simulink model "Controller_ABS_VLC_AYC"  (Simulink 8.7)
settings: Solver=ode3  SolverMode=SingleTasking  StartTime=0.0  StopTime=6  FixedStep=0.001  RelTol=1e-3
undefined symbols (not defined in the file): fdesignblkfcn, gcbh, Lf, Lr, T_Avail
libraries: fuzblock x17, simulink x8
(part 1 of 2)
settings Model: MinMaxOverflowLogging=ForceOff  Creator=MR Spyder  LastModifiedBy=kschmutz
settings DataIOCC: SignalLoggingSaveFormat=ModelDataLogs  SaveOutput=off  SaveTime=off
settings OptimizationCC: DefaultParameterBehavior=Inlined  ExpressionDepthLimit=2147483647
settings DebuggingCC: SolverPrmCheckMsg=warning  FcnCallInpInsideContextMsg=EnableAllAsWarning  StateNameClashWarn=warning
settings GRTTargetCC: CombineOutputUpdateFcns=off  GRTInterface=on

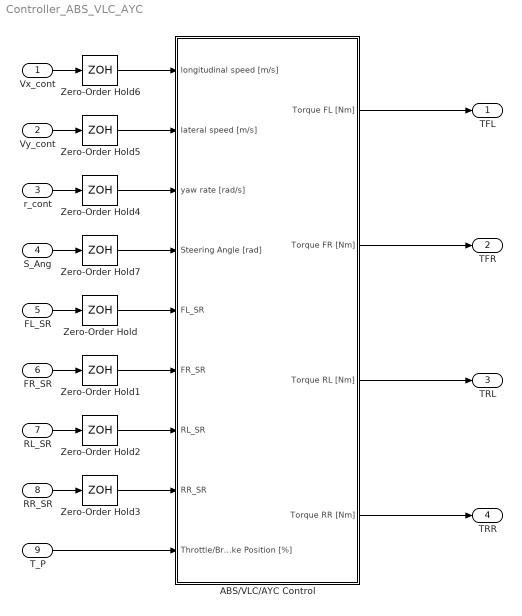
== system Controller_ABS_VLC_AYC ==
  Vx_cont : Inport
  Vy_cont : Inport  Port=2
  r_cont : Inport  Port=3
  S_Ang : Inport  Port=4
  FL_SR : Inport  Port=5
  FR_SR : Inport  Port=6
  RL_SR : Inport  Port=7
  RR_SR : Inport  Port=8
  T_P : Inport  Port=9
  ABS/VLC/AYC Control : Subsystem
  Zero-Order Hold{,1..7} (8 alike) : ZeroOrderHold  SampleTime=0.001
  TFL : Outport
  TFR : Outport  Port=2
  TRL : Outport  Port=3
  TRR : Outport  Port=4
  wires:
  Vx_cont/1 -> Zero-Order Hold6/1
  Vy_cont/1 -> Zero-Order Hold5/1
  r_cont/1 -> Zero-Order Hold4/1
  S_Ang/1 -> Zero-Order Hold7/1
  FL_SR/1 -> Zero-Order Hold/1
  FR_SR/1 -> Zero-Order Hold1/1
  RL_SR/1 -> Zero-Order Hold2/1
  RR_SR/1 -> Zero-Order Hold3/1
  T_P/1 -> ABS/VLC/AYC Control/9(Throttle/Brake Position [%])
  ABS/VLC/AYC Control/1(Torque FL [Nm]) -> TFL/1
  ABS/VLC/AYC Control/2(Torque FR [Nm]) -> TFR/1
  ABS/VLC/AYC Control/3(Torque RL [Nm]) -> TRL/1
  ABS/VLC/AYC Control/4(Torque RR [Nm]) -> TRR/1
  Zero-Order Hold/1 -> ABS/VLC/AYC Control/5(FL_SR)
  Zero-Order Hold1/1 -> ABS/VLC/AYC Control/6(FR_SR)
  Zero-Order Hold2/1 -> ABS/VLC/AYC Control/7(RL_SR)
  Zero-Order Hold3/1 -> ABS/VLC/AYC Control/8(RR_SR)
  Zero-Order Hold4/1 -> ABS/VLC/AYC Control/3(yaw rate [rad/s])
  Zero-Order Hold5/1 -> ABS/VLC/AYC Control/2(lateral speed [m/s])
  Zero-Order Hold6/1 -> ABS/VLC/AYC Control/1(longitudinal speed [m/s])
  Zero-Order Hold7/1 -> ABS/VLC/AYC Control/4(Steering Angle [rad])

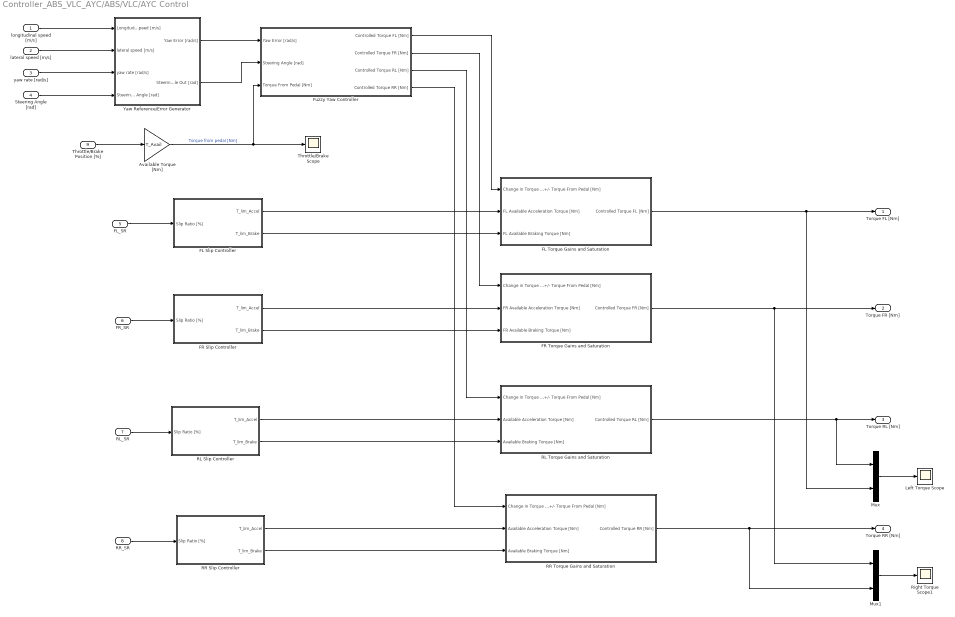
== system Controller_ABS_VLC_AYC/ABS/VLC/AYC Control ==
  longitudinal speed [m/s] : Inport
  lateral speed [m/s] : Inport  Port=2
  yaw rate [rad/s] : Inport  Port=3
  Steering Angle [rad] : Inport  Port=4
  FL_SR : Inport  Port=5
  FR_SR : Inport  Port=6
  RL_SR : Inport  Port=7
  RR_SR : Inport  Port=8
  Throttle/Brake Position [%] : Inport  Port=9
  Available Torque [Nm] : Gain  Gain=T_Avail
  FL Slip Controller : Subsystem
  FL Torque Gains and Saturation : Subsystem
  FR Slip Controller : Subsystem
  FR Torque Gains and Saturation : Subsystem
  Fuzzy Yaw Controller : Subsystem
  Left Torque Scope : Scope
  Mux : Mux  Inputs=2
  Mux1 : Mux  Inputs=2
  RL Slip Controller : Subsystem
  RL Torque Gains and Saturation : Subsystem
  RR Slip Controller : Subsystem
  RR Torque Gains and Saturation : Subsystem
  Right Torque Scope1 : Scope
  Throttle/Brake Scope : Scope
  Yaw Reference/Error Generator : Subsystem
  Torque FL [Nm] : Outport
  Torque FR [Nm] : Outport  Port=2
  Torque RL [Nm] : Outport  Port=3
  Torque RR [Nm] : Outport  Port=4
  wires:
  FL_SR/1 -> FL Slip Controller/1(Slip Ratio [%])
  Mux/1 -> Left Torque Scope/1
  longitudinal speed [m/s]/1 -> Yaw Reference/Error Generator/1(Longitudinal Speed [m/s])
  lateral speed [m/s]/1 -> Yaw Reference/Error Generator/2(lateral speed [m/s])
  yaw rate [rad/s]/1 -> Yaw Reference/Error Generator/3(yaw rate [rad/s])
  Steering Angle [rad]/1 -> Yaw Reference/Error Generator/4(Steering Angle [rad])
  Throttle/Brake Position [%]/1 -> Available Torque [Nm]/1
  Available Torque [Nm]/1 -> Fuzzy Yaw Controller/3(Torque From Pedal [Nm]), Throttle/Brake Scope/1  "Torque from pedal [Nm]"
  FL Slip Controller/1(T_lim_Accel) -> FL Torque Gains and Saturation/2(FL Available Acceleration Torque [Nm])
  FL Slip Controller/2(T_lim_Brake) -> FL Torque Gains and Saturation/3(FL Available Braking Torque [Nm])
  Yaw Reference/Error Generator/1(Yaw Error [rad/s]) -> Fuzzy Yaw Controller/1(Yaw Error [rad/s])
  Yaw Reference/Error Generator/2(Steering Angle Out [rad]) -> Fuzzy Yaw Controller/2(Steering Angle [rad])
  Fuzzy Yaw Controller/1(Controlled Torque FL [Nm]) -> FL Torque Gains and Saturation/1(Change in Torque +/- Torque From Pedal [Nm])
  Fuzzy Yaw Controller/2(Controlled Torque FR [Nm]) -> FR Torque Gains and Saturation/1(Change in Torque +/- Torque From Pedal [Nm])
  Fuzzy Yaw Controller/3(Controlled Torque RL [Nm]) -> RL Torque Gains and Saturation/1(Change in Torque +/- Torque From Pedal [Nm])
  Fuzzy Yaw Controller/4(Controlled Torque RR [Nm]) -> RR Torque Gains and Saturation/1(Change in Torque +/- Torque From Pedal [Nm])
  FL Torque Gains and Saturation/1(Controlled Torque FL [Nm]) -> Torque FL [Nm]/1, Mux/2
  FR Torque Gains and Saturation/1(Controlled Torque FR [Nm]) -> Torque FR [Nm]/1, Mux1/1
  RL Torque Gains and Saturation/1(Controlled Torque RL [Nm]) -> Torque RL [Nm]/1, Mux/1
  RR Torque Gains and Saturation/1(Controlled Torque RR [Nm]) -> Torque RR [Nm]/1, Mux1/2
  RL_SR/1 -> RL Slip Controller/1(Slip Ratio [%])
  RR_SR/1 -> RR Slip Controller/1(Slip Ratio [%])
  FR Slip Controller/1(T_lim_Accel) -> FR Torque Gains and Saturation/2(FR Available Acceleration Torque [Nm])
  FR Slip Controller/2(T_lim_Brake) -> FR Torque Gains and Saturation/3(FR Available Braking Torque [Nm])
  RL Slip Controller/1(T_lim_Accel) -> RL Torque Gains and Saturation/2(Available Acceleration Torque [Nm])
  RL Slip Controller/2(T_lim_Brake) -> RL Torque Gains and Saturation/3(Available Braking Torque [Nm])
  RR Slip Controller/1(T_lim_Accel) -> RR Torque Gains and Saturation/2(Available Acceleration Torque [Nm])
  RR Slip Controller/2(T_lim_Brake) -> RR Torque Gains and Saturation/3(Available Braking Torque [Nm])
  Mux1/1 -> Right Torque Scope1/1
  FR_SR/1 -> FR Slip Controller/1(Slip Ratio [%])

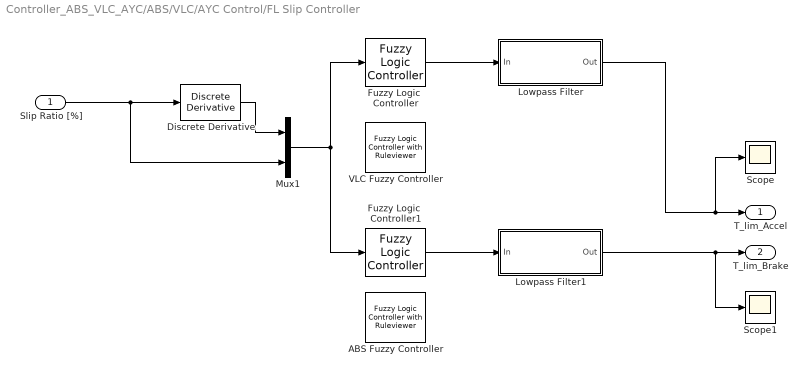
== system Controller_ABS_VLC_AYC/ABS/VLC/AYC Control/FL Slip Controller ==
  Slip Ratio [%] : Inport
  ABS Fuzzy Controller : fuzblock/Fuzzy Logic  Controller  with Ruleviewer  fismatrix=Fuzzy_Slip_Ctl_ABS  Ts=.1
  Discrete Derivative : simulink/Discrete/Discrete Derivative  gainval=1.0  ICPrevScaledInput=0.0  InputProcessing=Inherited  OutMin=[]  OutMax=[]  OutDataType=fixdt(1, 16)  OutScaling=2^-10  DoSatur=off
  Fuzzy Logic  Controller : fuzblock/Fuzzy Logic  Controller  fis=Fuzzy_Slip_Ctl_VLC
  Fuzzy Logic  Controller1 : fuzblock/Fuzzy Logic  Controller  fis=Fuzzy_Slip_Ctl_ABS
  Lowpass Filter : Subsystem  DialogController=fdesignblkfcn  DialogControllerArgs=DataTag1  InitFcn=fdesignblkfcn(gcbh, {'InitFcn'});  mask(Lowpass Filter){}
      mask help: Design a lowpass filter
      settings: CopyFcn=fdesignblkfcn(gcbh, {'CopyFcn'});
      mask Help: helpview(mapfilelocation('dsp'), 'dsplowpassfilter');
      mask Display: disp('Lowpass')
  Lowpass Filter1 : Subsystem  DialogController=fdesignblkfcn  DialogControllerArgs=DataTag3  InitFcn=fdesignblkfcn(gcbh, {'InitFcn'});  mask(Lowpass Filter){}
      mask help: Design a lowpass filter
      settings: CopyFcn=fdesignblkfcn(gcbh, {'CopyFcn'});
      mask Help: helpview(mapfilelocation('dsp'), 'dsplowpassfilter');
      mask Display: disp('Lowpass')
  Mux1 : Mux  Inputs=2
  Scope : Scope
  Scope1 : Scope
  VLC Fuzzy Controller : fuzblock/Fuzzy Logic  Controller  with Ruleviewer  fismatrix=Fuzzy_Slip_Ctl_VLC  Ts=.1
  T_lim_Accel : Outport
  T_lim_Brake : Outport  Port=2
  wires:
  Mux1/1 -> Fuzzy Logic  Controller/1, Fuzzy Logic  Controller1/1
  Slip Ratio [%]/1 -> Mux1/2, Discrete Derivative/1
  Discrete Derivative/1 -> Mux1/1
  Fuzzy Logic  Controller/1 -> Lowpass Filter/1(In)
  Fuzzy Logic  Controller1/1 -> Lowpass Filter1/1(In)
  Lowpass Filter/1(Out) -> T_lim_Accel/1, Scope/1
  Lowpass Filter1/1(Out) -> T_lim_Brake/1, Scope1/1

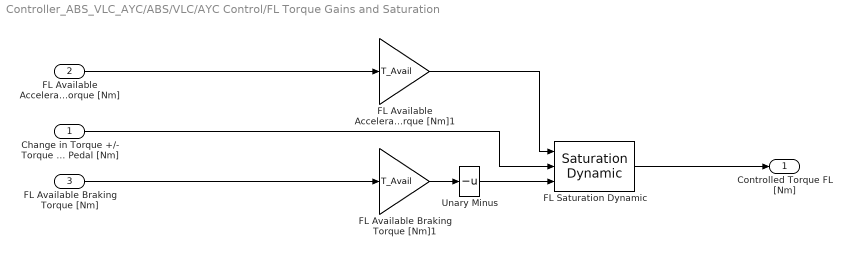
== system Controller_ABS_VLC_AYC/ABS/VLC/AYC Control/FL Torque Gains and Saturation ==
  Change in Torque +/- Torque From Pedal [Nm] : Inport
  FL Available Acceleration Torque [Nm] : Inport  Port=2
  FL Available Braking Torque [Nm] : Inport  Port=3
  FL Available Acceleration Torque [Nm]1 : Gain  Gain=T_Avail
  FL Available Braking Torque [Nm]1 : Gain  Gain=T_Avail
  FL Saturation Dynamic : simulink/Discontinuities/Saturation Dynamic  OutMin=[]  OutMax=[]  OutDataTypeStr=Inherit: Same as second input  OutDataType=fixdt(1, 16)  OutScaling=2^-10  DoSatur=off
  Unary Minus : UnaryMinus
  Controlled Torque FL [Nm] : Outport
  wires:
  FL Available Acceleration Torque [Nm]1/1 -> FL Saturation Dynamic/1
  Unary Minus/1 -> FL Saturation Dynamic/3
  FL Available Braking Torque [Nm]1/1 -> Unary Minus/1
  FL Available Acceleration Torque [Nm]/1 -> FL Available Acceleration Torque [Nm]1/1
  FL Available Braking Torque [Nm]/1 -> FL Available Braking Torque [Nm]1/1
  Change in Torque +/- Torque From Pedal [Nm]/1 -> FL Saturation Dynamic/2
  FL Saturation Dynamic/1 -> Controlled Torque FL [Nm]/1

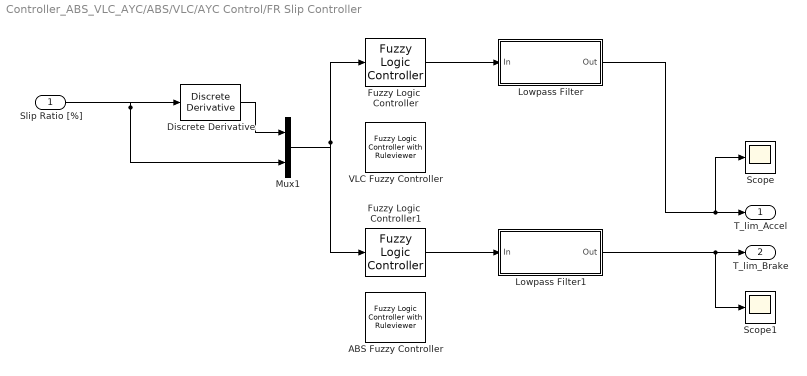
== system Controller_ABS_VLC_AYC/ABS/VLC/AYC Control/FR Slip Controller ==
  Slip Ratio [%] : Inport
  ABS Fuzzy Controller : fuzblock/Fuzzy Logic  Controller  with Ruleviewer  fismatrix=Fuzzy_Slip_Ctl_ABS  Ts=.1
  Discrete Derivative : simulink/Discrete/Discrete Derivative  gainval=1.0  ICPrevScaledInput=0.0  InputProcessing=Inherited  OutMin=[]  OutMax=[]  OutDataType=fixdt(1, 16)  OutScaling=2^-10  DoSatur=off
  Fuzzy Logic  Controller : fuzblock/Fuzzy Logic  Controller  fis=Fuzzy_Slip_Ctl_VLC
  Fuzzy Logic  Controller1 : fuzblock/Fuzzy Logic  Controller  fis=Fuzzy_Slip_Ctl_ABS
  Lowpass Filter : Subsystem  DialogController=fdesignblkfcn  DialogControllerArgs=DataTag5  InitFcn=fdesignblkfcn(gcbh, {'InitFcn'});  mask(Lowpass Filter){}
      mask help: Design a lowpass filter
      settings: CopyFcn=fdesignblkfcn(gcbh, {'CopyFcn'});
      mask Help: helpview(mapfilelocation('dsp'), 'dsplowpassfilter');
      mask Display: disp('Lowpass')
  Lowpass Filter1 : Subsystem  DialogController=fdesignblkfcn  DialogControllerArgs=DataTag7  InitFcn=fdesignblkfcn(gcbh, {'InitFcn'});  mask(Lowpass Filter){}
      mask help: Design a lowpass filter
      settings: CopyFcn=fdesignblkfcn(gcbh, {'CopyFcn'});
      mask Help: helpview(mapfilelocation('dsp'), 'dsplowpassfilter');
      mask Display: disp('Lowpass')
  Mux1 : Mux  Inputs=2
  Scope : Scope
  Scope1 : Scope
  VLC Fuzzy Controller : fuzblock/Fuzzy Logic  Controller  with Ruleviewer  fismatrix=Fuzzy_Slip_Ctl_VLC  Ts=.1
  T_lim_Accel : Outport
  T_lim_Brake : Outport  Port=2
  wires:
  Mux1/1 -> Fuzzy Logic  Controller/1, Fuzzy Logic  Controller1/1
  Slip Ratio [%]/1 -> Mux1/2, Discrete Derivative/1
  Discrete Derivative/1 -> Mux1/1
  Fuzzy Logic  Controller/1 -> Lowpass Filter/1(In)
  Fuzzy Logic  Controller1/1 -> Lowpass Filter1/1(In)
  Lowpass Filter/1(Out) -> T_lim_Accel/1, Scope/1
  Lowpass Filter1/1(Out) -> T_lim_Brake/1, Scope1/1

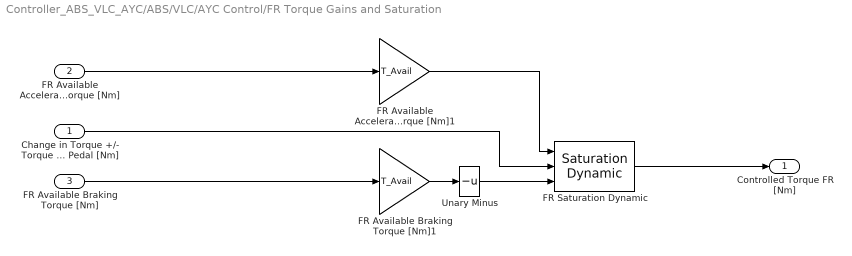
== system Controller_ABS_VLC_AYC/ABS/VLC/AYC Control/FR Torque Gains and Saturation ==
  Change in Torque +/- Torque From Pedal [Nm] : Inport
  FR Available Acceleration Torque [Nm] : Inport  Port=2
  FR Available Braking Torque [Nm] : Inport  Port=3
  FR Available Acceleration Torque [Nm]1 : Gain  Gain=T_Avail
  FR Available Braking Torque [Nm]1 : Gain  Gain=T_Avail
  FR Saturation Dynamic : simulink/Discontinuities/Saturation Dynamic  OutMin=[]  OutMax=[]  OutDataTypeStr=Inherit: Same as second input  OutDataType=fixdt(1, 16)  OutScaling=2^-10  DoSatur=off
  Unary Minus : UnaryMinus
  Controlled Torque FR [Nm] : Outport
  wires:
  FR Available Acceleration Torque [Nm]1/1 -> FR Saturation Dynamic/1
  Unary Minus/1 -> FR Saturation Dynamic/3
  FR Available Braking Torque [Nm]1/1 -> Unary Minus/1
  FR Available Acceleration Torque [Nm]/1 -> FR Available Acceleration Torque [Nm]1/1
  FR Available Braking Torque [Nm]/1 -> FR Available Braking Torque [Nm]1/1
  Change in Torque +/- Torque From Pedal [Nm]/1 -> FR Saturation Dynamic/2
  FR Saturation Dynamic/1 -> Controlled Torque FR [Nm]/1

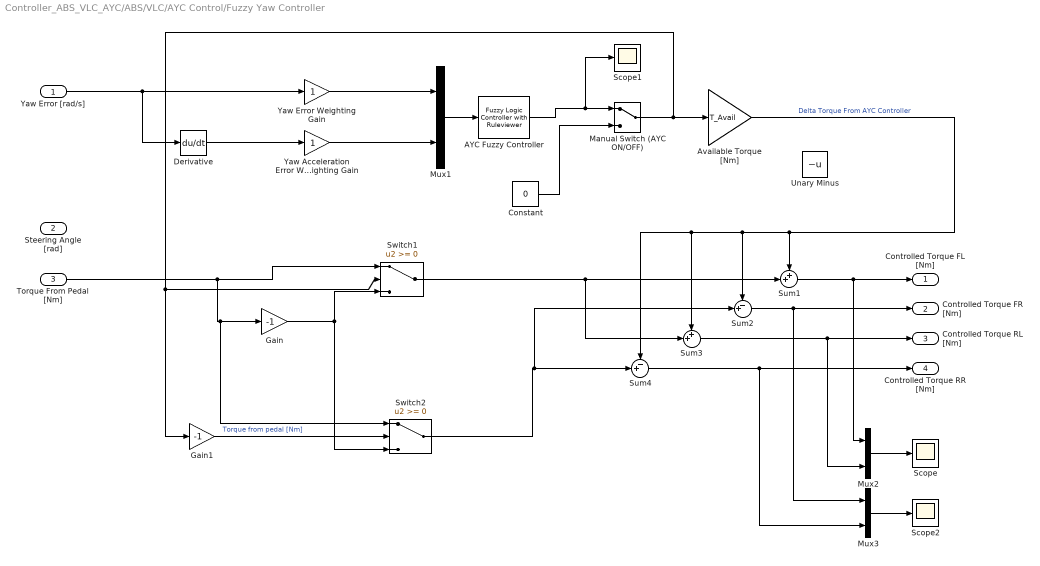
== system Controller_ABS_VLC_AYC/ABS/VLC/AYC Control/Fuzzy Yaw Controller ==
  Yaw Error [rad/s] : Inport
  Steering Angle [rad] : Inport  Port=2
  Torque From Pedal [Nm] : Inport  Port=3
  AYC Fuzzy Controller : fuzblock/Fuzzy Logic  Controller  with Ruleviewer  fismatrix=Fuzzy_AYC_Ctl  Ts=.1
  Available Torque [Nm] : Gain  Gain=T_Avail
  Constant : Constant  Value=0
  Derivative : Derivative
  Gain : Gain  Gain=-1
  Gain1 : Gain  Gain=-1
  Manual Switch (AYC ON/OFF) : ManualSwitch
  Mux1 : Mux  Inputs=2
  Mux2 : Mux  Inputs=2
  Mux3 : Mux  Inputs=2
  Scope : Scope
  Scope1 : Scope
  Scope2 : Scope
  Sum1 : Sum  Inputs=++|
  Sum2 : Sum  Inputs=-+|
  Sum3 : Sum  Inputs=++|
  Sum4 : Sum  Inputs=-+|
  Switch1 : Switch
  Switch2 : Switch
  Unary Minus : UnaryMinus
  Yaw Acceleration Error Weighting Gain : Gain
  Yaw Error Weighting Gain : Gain
  Controlled Torque FL [Nm] : Outport
  Controlled Torque FR [Nm] : Outport  Port=2
  Controlled Torque RL [Nm] : Outport  Port=3
  Controlled Torque RR [Nm] : Outport  Port=4
  wires:
  Sum1/1 -> Controlled Torque FL [Nm]/1, Mux2/1
  Sum2/1 -> Controlled Torque FR [Nm]/1, Mux3/1
  Sum3/1 -> Controlled Torque RL [Nm]/1, Mux2/2
  Sum4/1 -> Controlled Torque RR [Nm]/1, Mux3/2
  Mux1/1 -> AYC Fuzzy Controller/1
  Yaw Error [rad/s]/1 -> Yaw Error Weighting Gain/1, Derivative/1
  Yaw Error Weighting Gain/1 -> Mux1/1
  Yaw Acceleration Error Weighting Gain/1 -> Mux1/2
  Mux2/1 -> Scope/1
  AYC Fuzzy Controller/1 -> Manual Switch (AYC ON/OFF)/1, Scope1/1
  Constant/1 -> Manual Switch (AYC ON/OFF)/2
  Manual Switch (AYC ON/OFF)/1 -> Gain1/1, Switch1/2, Available Torque [Nm]/1
  Mux3/1 -> Scope2/1
  Available Torque [Nm]/1 -> Sum4/1, Sum3/1, Sum2/1, Sum1/1  "Delta Torque From AYC Controller"
  Derivative/1 -> Yaw Acceleration Error Weighting Gain/1
  Switch1/1 -> Sum3/2, Sum1/2
  Gain/1 -> Switch2/3, Switch1/3
  Torque From Pedal [Nm]/1 -> Switch2/1, Gain/1, Switch1/1  "Torque from pedal [Nm]"
  Switch2/1 -> Sum2/2, Sum4/2
  Gain1/1 -> Switch2/2

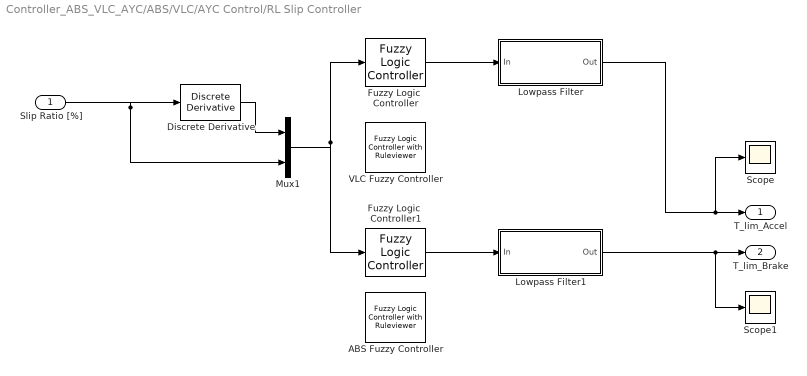
== system Controller_ABS_VLC_AYC/ABS/VLC/AYC Control/RL Slip Controller ==
  Slip Ratio [%] : Inport
  ABS Fuzzy Controller : fuzblock/Fuzzy Logic  Controller  with Ruleviewer  fismatrix=Fuzzy_Slip_Ctl_ABS  Ts=.1
  Discrete Derivative : simulink/Discrete/Discrete Derivative  gainval=1.0  ICPrevScaledInput=0.0  InputProcessing=Inherited  OutMin=[]  OutMax=[]  OutDataType=fixdt(1, 16)  OutScaling=2^-10  DoSatur=off
  Fuzzy Logic  Controller : fuzblock/Fuzzy Logic  Controller  fis=Fuzzy_Slip_Ctl_VLC
  Fuzzy Logic  Controller1 : fuzblock/Fuzzy Logic  Controller  fis=Fuzzy_Slip_Ctl_ABS
  Lowpass Filter : Subsystem  DialogController=fdesignblkfcn  DialogControllerArgs=DataTag9  InitFcn=fdesignblkfcn(gcbh, {'InitFcn'});  mask(Lowpass Filter){}
      mask help: Design a lowpass filter
      settings: CopyFcn=fdesignblkfcn(gcbh, {'CopyFcn'});
      mask Help: helpview(mapfilelocation('dsp'), 'dsplowpassfilter');
      mask Display: disp('Lowpass')
  Lowpass Filter1 : Subsystem  DialogController=fdesignblkfcn  DialogControllerArgs=DataTag11  InitFcn=fdesignblkfcn(gcbh, {'InitFcn'});  mask(Lowpass Filter){}
      mask help: Design a lowpass filter
      settings: CopyFcn=fdesignblkfcn(gcbh, {'CopyFcn'});
      mask Help: helpview(mapfilelocation('dsp'), 'dsplowpassfilter');
      mask Display: disp('Lowpass')
  Mux1 : Mux  Inputs=2
  Scope : Scope
  Scope1 : Scope
  VLC Fuzzy Controller : fuzblock/Fuzzy Logic  Controller  with Ruleviewer  fismatrix=Fuzzy_Slip_Ctl_VLC  Ts=.1
  T_lim_Accel : Outport
  T_lim_Brake : Outport  Port=2
  wires:
  Mux1/1 -> Fuzzy Logic  Controller/1, Fuzzy Logic  Controller1/1
  Slip Ratio [%]/1 -> Mux1/2, Discrete Derivative/1
  Discrete Derivative/1 -> Mux1/1
  Fuzzy Logic  Controller/1 -> Lowpass Filter/1(In)
  Fuzzy Logic  Controller1/1 -> Lowpass Filter1/1(In)
  Lowpass Filter/1(Out) -> T_lim_Accel/1, Scope/1
  Lowpass Filter1/1(Out) -> T_lim_Brake/1, Scope1/1

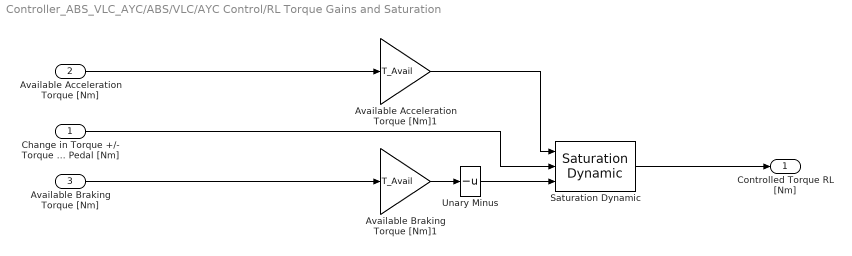
== system Controller_ABS_VLC_AYC/ABS/VLC/AYC Control/RL Torque Gains and Saturation ==
  Change in Torque +/- Torque From Pedal [Nm] : Inport
  Available Acceleration Torque [Nm] : Inport  Port=2
  Available Braking Torque [Nm] : Inport  Port=3
  Available Acceleration Torque [Nm]1 : Gain  Gain=T_Avail
  Available Braking Torque [Nm]1 : Gain  Gain=T_Avail
  Saturation Dynamic : simulink/Discontinuities/Saturation Dynamic  OutMin=[]  OutMax=[]  OutDataTypeStr=Inherit: Same as second input  OutDataType=fixdt(1, 16)  OutScaling=2^-10  DoSatur=off
  Unary Minus : UnaryMinus
  Controlled Torque RL [Nm] : Outport
  wires:
  Available Acceleration Torque [Nm]1/1 -> Saturation Dynamic/1
  Unary Minus/1 -> Saturation Dynamic/3
  Available Braking Torque [Nm]1/1 -> Unary Minus/1
  Available Acceleration Torque [Nm]/1 -> Available Acceleration Torque [Nm]1/1
  Available Braking Torque [Nm]/1 -> Available Braking Torque [Nm]1/1
  Change in Torque +/- Torque From Pedal [Nm]/1 -> Saturation Dynamic/2
  Saturation Dynamic/1 -> Controlled Torque RL [Nm]/1

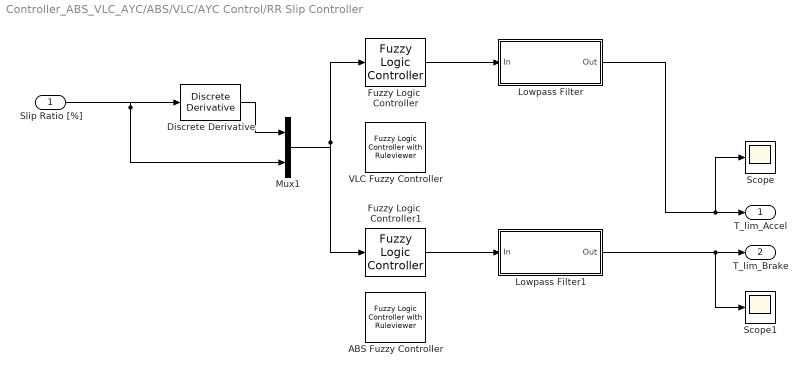
== system Controller_ABS_VLC_AYC/ABS/VLC/AYC Control/RR Slip Controller ==
  Slip Ratio [%] : Inport
  ABS Fuzzy Controller : fuzblock/Fuzzy Logic  Controller  with Ruleviewer  fismatrix=Fuzzy_Slip_Ctl_ABS  Ts=.1
  Discrete Derivative : simulink/Discrete/Discrete Derivative  gainval=1.0  ICPrevScaledInput=0.0  InputProcessing=Inherited  OutMin=[]  OutMax=[]  OutDataType=fixdt(1, 16)  OutScaling=2^-10  DoSatur=off
  Fuzzy Logic  Controller : fuzblock/Fuzzy Logic  Controller  fis=Fuzzy_Slip_Ctl_VLC
  Fuzzy Logic  Controller1 : fuzblock/Fuzzy Logic  Controller  fis=Fuzzy_Slip_Ctl_ABS
  Lowpass Filter : Subsystem  DialogController=fdesignblkfcn  DialogControllerArgs=DataTag13  InitFcn=fdesignblkfcn(gcbh, {'InitFcn'});  mask(Lowpass Filter){}
      mask help: Design a lowpass filter
      settings: CopyFcn=fdesignblkfcn(gcbh, {'CopyFcn'});
      mask Help: helpview(mapfilelocation('dsp'), 'dsplowpassfilter');
      mask Display: disp('Lowpass')
  Lowpass Filter1 : Subsystem  DialogController=fdesignblkfcn  DialogControllerArgs=DataTag15  InitFcn=fdesignblkfcn(gcbh, {'InitFcn'});  mask(Lowpass Filter){}
      mask help: Design a lowpass filter
      settings: CopyFcn=fdesignblkfcn(gcbh, {'CopyFcn'});
      mask Help: helpview(mapfilelocation('dsp'), 'dsplowpassfilter');
      mask Display: disp('Lowpass')
  Mux1 : Mux  Inputs=2
  Scope : Scope
  Scope1 : Scope
  VLC Fuzzy Controller : fuzblock/Fuzzy Logic  Controller  with Ruleviewer  fismatrix=Fuzzy_Slip_Ctl_VLC  Ts=.1
  T_lim_Accel : Outport
  T_lim_Brake : Outport  Port=2
  wires:
  Mux1/1 -> Fuzzy Logic  Controller/1, Fuzzy Logic  Controller1/1
  Slip Ratio [%]/1 -> Mux1/2, Discrete Derivative/1
  Discrete Derivative/1 -> Mux1/1
  Fuzzy Logic  Controller/1 -> Lowpass Filter/1(In)
  Fuzzy Logic  Controller1/1 -> Lowpass Filter1/1(In)
  Lowpass Filter/1(Out) -> T_lim_Accel/1, Scope/1
  Lowpass Filter1/1(Out) -> T_lim_Brake/1, Scope1/1

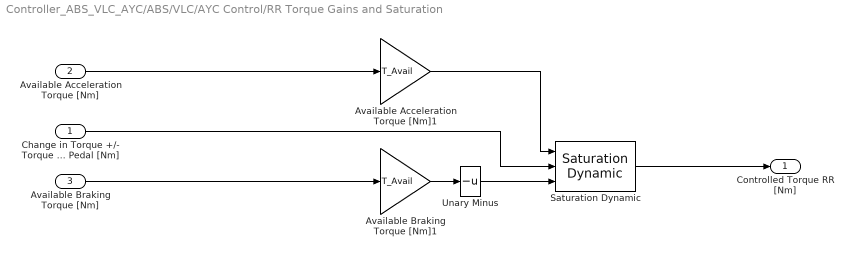
== system Controller_ABS_VLC_AYC/ABS/VLC/AYC Control/RR Torque Gains and Saturation ==
  Change in Torque +/- Torque From Pedal [Nm] : Inport
  Available Acceleration Torque [Nm] : Inport  Port=2
  Available Braking Torque [Nm] : Inport  Port=3
  Available Acceleration Torque [Nm]1 : Gain  Gain=T_Avail
  Available Braking Torque [Nm]1 : Gain  Gain=T_Avail
  Saturation Dynamic : simulink/Discontinuities/Saturation Dynamic  OutMin=[]  OutMax=[]  OutDataTypeStr=Inherit: Same as second input  OutDataType=fixdt(1, 16)  OutScaling=2^-10  DoSatur=off
  Unary Minus : UnaryMinus
  Controlled Torque RR [Nm] : Outport
  wires:
  Available Acceleration Torque [Nm]1/1 -> Saturation Dynamic/1
  Unary Minus/1 -> Saturation Dynamic/3
  Available Braking Torque [Nm]1/1 -> Unary Minus/1
  Available Acceleration Torque [Nm]/1 -> Available Acceleration Torque [Nm]1/1
  Available Braking Torque [Nm]/1 -> Available Braking Torque [Nm]1/1
  Change in Torque +/- Torque From Pedal [Nm]/1 -> Saturation Dynamic/2
  Saturation Dynamic/1 -> Controlled Torque RR [Nm]/1

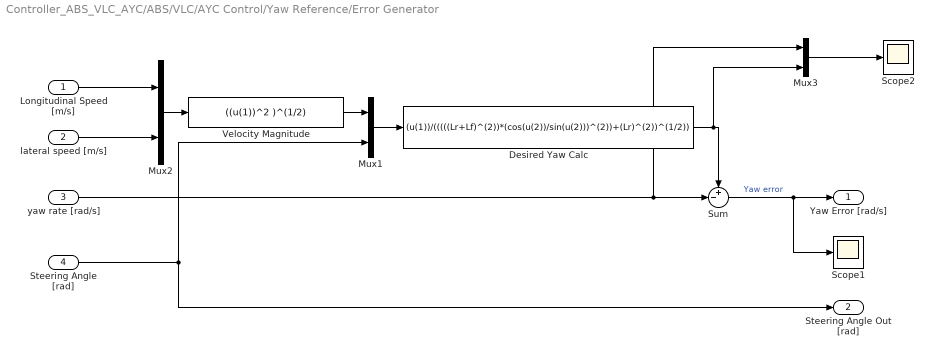
== system Controller_ABS_VLC_AYC/ABS/VLC/AYC Control/Yaw Reference/Error Generator ==
  Longitudinal Speed [m/s] : Inport
  lateral speed [m/s] : Inport  Port=2
  yaw rate [rad/s] : Inport  Port=3
  Steering Angle [rad] : Inport  Port=4
  Desired Yaw Calc : Fcn  Expr=(u(1))/(((((Lr+Lf)^(2))*(cos(u(2))/sin(u(2)))^(2))+(Lr)^(2))^(1/2))
  Mux1 : Mux  Inputs=2
  Mux2 : Mux  Inputs=2
  Mux3 : Mux  Inputs=2
  Scope1 : Scope
  Scope2 : Scope
  Sum : Sum  Inputs=+-|
  Velocity Magnitude : Fcn  Expr=((u(1))^2 )^(1/2)
  Yaw Error [rad/s] : Outport
  Steering Angle Out [rad] : Outport  Port=2
  wires:
  Mux1/1 -> Desired Yaw Calc/1
  lateral speed [m/s]/1 -> Mux2/2
  Longitudinal Speed [m/s]/1 -> Mux2/1
  Mux2/1 -> Velocity Magnitude/1
  Velocity Magnitude/1 -> Mux1/1
  Steering Angle [rad]/1 -> Mux1/2, Steering Angle Out [rad]/1
  yaw rate [rad/s]/1 -> Sum/2, Mux3/1
  Desired Yaw Calc/1 -> Sum/1, Mux3/2
  Sum/1 -> Yaw Error [rad/s]/1, Scope1/1  "Yaw error"
  Mux3/1 -> Scope2/1

== system Controller_ABS_VLC_AYC/ABS/VLC/AYC Control/FL Slip Controller/Lowpass Filter ==
  In : Inport
  Generated Filter Block : DiscreteFir  Tag=BlockMethodSubSystem  Coefficients=[-0.00075646864062919763 -0.00063948505713481811 -0.00086554492949518676 -0.0011037990733813235 -0.001339284284868959 -0.0015547400053551874 -0.0017300944700606284 -0.00184670274387296 -0.0018881302599738493 -0.0018383815937568033 -0.0016908823878034785 -0.0014415887943325673 -0.0010961195158699811 -0.00066631717319359861 -0.00017121409252519941 0.00036359936416717264 0.0009080465739429777 0.0014298736348337699 0.0018960211364896008 0.0022771863603771665 0.0025482618478869408 0.002692222556903226 0.0027008445578628891 0.0025759682427628858 0.0023298680220744062 0.001984391370697888 0.0015692141720698332 0.0011200194544684224 0.00067461876056971635 0.00027061032753731694 -5.866179415617268e-05 -0.00028669635689133085 -0.00039633166387144857 -0.00038148906017572019 -0.0002477702828760265 -1.1936356441557194e-05 0.00029922490683921712 0.00065189802033198212 0.0010079363042756382 0.0013289590517563921 0.0015799187563950311 0.001732598437530234 0.0017685449960751973 0.0016809867202291359 0.001475577844518795 0.0011702671086116819 0.00079334294519489744 0.00038107291302585564 -2.6111427728838237e-05 -0.00038757608995898589 -0.00066664955030768121 -0.00083452345222956249 -0.0008733550143161324 -0.00077824476354573693 -0.00055819296971255797 -0.00023521601512397369 0.00015742126605453337 0.0005785784851626923 0.00098328250386749182 0.0013273087132983671 0.0015718484935428579 0.0016876773286742383 0.0016583648153362584 0.0014824517181836361 0.001173793218361215 0.00076066718725827424 0.00028306324114901494 -0.00021118635508748061 -0.00067122011711513783 -0.0010484581457023382 -0.0013017758532885772 -0.0014019618554660471 -0.0013352201239705105 -0.0011048842486169792 -0.00073165621411404097 -0.00025182527315658872 0.00028610350920870874 0.00082615867146424533 0.0013106234674959305 0.0016860834546990108 0.0019091311706072877 0.0019513306436192534 0.0018025262485976861 0.0014725312016039653 0.00099060478772183152 0.00040292530986260334 -0.00023178098881511844 -0.00084810728175012385 -0.0013806963630004151 -0.0017711026206815544 -0.0019742574925858663 -0.0019635291020280035 -0.0017341538241868613 -0.0013043450108582717 -0.00071404805444023607 -2.1386504594989465e-05 0.00070295843642983579 0.0013828574770577515 0.0019445780369022776 0.0023247321243138005 0.0024772174699799845 0.0023786792654153892 0.0020316457847079574 0.0014650458441179052 0.00073198021892930624 -9.5165616451746313e-05 -0.00093179550640667356 -0.0016896353737900064 -0.002286029399938193 -0.0026528026156592069 -0.0027439824010879752 -0.0025413474050266682 -0.0020572239101028095 -0.0013341713539966283 -0.00044143094406244902 0.00053155699309554165 0.0014839255272411029 0.0023137406585026126 0.0029286981481292974 0.0032562467484617786 0.003251908926443922 0.0029049085085457831 0.0022404564981489922 0.0013182816267311918 0.00022746308219447748 -0.00092196135663783645 -0.0020099732300794516 -0.0029188826132397309 -0.0035458920722500759 -0.0038144882122502053 -0.0036834454103191363 -0.0031524540265802821 -0.0022636032725808913 -0.001098441233437557 0.00022918138522259228 0.0015840095633793522 0.0028228488017388279 0.0038094256961896428 0.0044290486254589569 0.0046015294833341713 0.0042909951378952392 0.0035113829579288443 0.002326900465678434 0.00084726356737852785 -0.00078210688654584614 -0.0023939506744333323 -0.0038159332671489276 -0.0048886091342003283 -0.0054827496552296451 -0.0055142584805278339 -0.0049549620495624256 -0.0038379957384760514 -0.0022570524748253273 -0.00035920054838253909 0.0016681240381698865 0.0036149620582436124 0.0052698289441135563 0.0064418143583644455 0.0069816111699239911 0.0067991979917402107 0.0058762117387505652 0.0042715432406493607 0.0021191551611802598 -0.00038190594776891601 -0.0029847547360424441 -0.0054177398262781288 -0.0074112614644437011 -0.0087258737465600832 -0.0091788423919074678 -0.0086664128929747897 -0.0071793804592940056 -0.004809945117289164 -0.0017488049914463934 0.0017278402015994767 0.0052806440695748677 0.0085371287675241395 ...(+5120 chars)]  InputProcessing=Columns as channels (frame based)
  Out : Outport
  wires:
  In/1 -> Generated Filter Block/1
  Generated Filter Block/1 -> Out/1

== system Controller_ABS_VLC_AYC/ABS/VLC/AYC Control/FL Slip Controller/Lowpass Filter1 ==
  In : Inport
  Generated Filter Block : DiscreteFir  Tag=BlockMethodSubSystem  Coefficients=[-0.00075646864062919763 -0.00063948505713481811 -0.00086554492949518676 -0.0011037990733813235 -0.001339284284868959 -0.0015547400053551874 -0.0017300944700606284 -0.00184670274387296 -0.0018881302599738493 -0.0018383815937568033 -0.0016908823878034785 -0.0014415887943325673 -0.0010961195158699811 -0.00066631717319359861 -0.00017121409252519941 0.00036359936416717264 0.0009080465739429777 0.0014298736348337699 0.0018960211364896008 0.0022771863603771665 0.0025482618478869408 0.002692222556903226 0.0027008445578628891 0.0025759682427628858 0.0023298680220744062 0.001984391370697888 0.0015692141720698332 0.0011200194544684224 0.00067461876056971635 0.00027061032753731694 -5.866179415617268e-05 -0.00028669635689133085 -0.00039633166387144857 -0.00038148906017572019 -0.0002477702828760265 -1.1936356441557194e-05 0.00029922490683921712 0.00065189802033198212 0.0010079363042756382 0.0013289590517563921 0.0015799187563950311 0.001732598437530234 0.0017685449960751973 0.0016809867202291359 0.001475577844518795 0.0011702671086116819 0.00079334294519489744 0.00038107291302585564 -2.6111427728838237e-05 -0.00038757608995898589 -0.00066664955030768121 -0.00083452345222956249 -0.0008733550143161324 -0.00077824476354573693 -0.00055819296971255797 -0.00023521601512397369 0.00015742126605453337 0.0005785784851626923 0.00098328250386749182 0.0013273087132983671 0.0015718484935428579 0.0016876773286742383 0.0016583648153362584 0.0014824517181836361 0.001173793218361215 0.00076066718725827424 0.00028306324114901494 -0.00021118635508748061 -0.00067122011711513783 -0.0010484581457023382 -0.0013017758532885772 -0.0014019618554660471 -0.0013352201239705105 -0.0011048842486169792 -0.00073165621411404097 -0.00025182527315658872 0.00028610350920870874 0.00082615867146424533 0.0013106234674959305 0.0016860834546990108 0.0019091311706072877 0.0019513306436192534 0.0018025262485976861 0.0014725312016039653 0.00099060478772183152 0.00040292530986260334 -0.00023178098881511844 -0.00084810728175012385 -0.0013806963630004151 -0.0017711026206815544 -0.0019742574925858663 -0.0019635291020280035 -0.0017341538241868613 -0.0013043450108582717 -0.00071404805444023607 -2.1386504594989465e-05 0.00070295843642983579 0.0013828574770577515 0.0019445780369022776 0.0023247321243138005 0.0024772174699799845 0.0023786792654153892 0.0020316457847079574 0.0014650458441179052 0.00073198021892930624 -9.5165616451746313e-05 -0.00093179550640667356 -0.0016896353737900064 -0.002286029399938193 -0.0026528026156592069 -0.0027439824010879752 -0.0025413474050266682 -0.0020572239101028095 -0.0013341713539966283 -0.00044143094406244902 0.00053155699309554165 0.0014839255272411029 0.0023137406585026126 0.0029286981481292974 0.0032562467484617786 0.003251908926443922 0.0029049085085457831 0.0022404564981489922 0.0013182816267311918 0.00022746308219447748 -0.00092196135663783645 -0.0020099732300794516 -0.0029188826132397309 -0.0035458920722500759 -0.0038144882122502053 -0.0036834454103191363 -0.0031524540265802821 -0.0022636032725808913 -0.001098441233437557 0.00022918138522259228 0.0015840095633793522 0.0028228488017388279 0.0038094256961896428 0.0044290486254589569 0.0046015294833341713 0.0042909951378952392 0.0035113829579288443 0.002326900465678434 0.00084726356737852785 -0.00078210688654584614 -0.0023939506744333323 -0.0038159332671489276 -0.0048886091342003283 -0.0054827496552296451 -0.0055142584805278339 -0.0049549620495624256 -0.0038379957384760514 -0.0022570524748253273 -0.00035920054838253909 0.0016681240381698865 0.0036149620582436124 0.0052698289441135563 0.0064418143583644455 0.0069816111699239911 0.0067991979917402107 0.0058762117387505652 0.0042715432406493607 0.0021191551611802598 -0.00038190594776891601 -0.0029847547360424441 -0.0054177398262781288 -0.0074112614644437011 -0.0087258737465600832 -0.0091788423919074678 -0.0086664128929747897 -0.0071793804592940056 -0.004809945117289164 -0.0017488049914463934 0.0017278402015994767 0.0052806440695748677 0.0085371287675241395 ...(+5120 chars)]  InputProcessing=Columns as channels (frame based)
  Out : Outport
  wires:
  In/1 -> Generated Filter Block/1
  Generated Filter Block/1 -> Out/1

== system Controller_ABS_VLC_AYC/ABS/VLC/AYC Control/FR Slip Controller/Lowpass Filter ==
  In : Inport
  Generated Filter Block : DiscreteFir  Tag=BlockMethodSubSystem  Coefficients=[-0.00075646864062919763 -0.00063948505713481811 -0.00086554492949518676 -0.0011037990733813235 -0.001339284284868959 -0.0015547400053551874 -0.0017300944700606284 -0.00184670274387296 -0.0018881302599738493 -0.0018383815937568033 -0.0016908823878034785 -0.0014415887943325673 -0.0010961195158699811 -0.00066631717319359861 -0.00017121409252519941 0.00036359936416717264 0.0009080465739429777 0.0014298736348337699 0.0018960211364896008 0.0022771863603771665 0.0025482618478869408 0.002692222556903226 0.0027008445578628891 0.0025759682427628858 0.0023298680220744062 0.001984391370697888 0.0015692141720698332 0.0011200194544684224 0.00067461876056971635 0.00027061032753731694 -5.866179415617268e-05 -0.00028669635689133085 -0.00039633166387144857 -0.00038148906017572019 -0.0002477702828760265 -1.1936356441557194e-05 0.00029922490683921712 0.00065189802033198212 0.0010079363042756382 0.0013289590517563921 0.0015799187563950311 0.001732598437530234 0.0017685449960751973 0.0016809867202291359 0.001475577844518795 0.0011702671086116819 0.00079334294519489744 0.00038107291302585564 -2.6111427728838237e-05 -0.00038757608995898589 -0.00066664955030768121 -0.00083452345222956249 -0.0008733550143161324 -0.00077824476354573693 -0.00055819296971255797 -0.00023521601512397369 0.00015742126605453337 0.0005785784851626923 0.00098328250386749182 0.0013273087132983671 0.0015718484935428579 0.0016876773286742383 0.0016583648153362584 0.0014824517181836361 0.001173793218361215 0.00076066718725827424 0.00028306324114901494 -0.00021118635508748061 -0.00067122011711513783 -0.0010484581457023382 -0.0013017758532885772 -0.0014019618554660471 -0.0013352201239705105 -0.0011048842486169792 -0.00073165621411404097 -0.00025182527315658872 0.00028610350920870874 0.00082615867146424533 0.0013106234674959305 0.0016860834546990108 0.0019091311706072877 0.0019513306436192534 0.0018025262485976861 0.0014725312016039653 0.00099060478772183152 0.00040292530986260334 -0.00023178098881511844 -0.00084810728175012385 -0.0013806963630004151 -0.0017711026206815544 -0.0019742574925858663 -0.0019635291020280035 -0.0017341538241868613 -0.0013043450108582717 -0.00071404805444023607 -2.1386504594989465e-05 0.00070295843642983579 0.0013828574770577515 0.0019445780369022776 0.0023247321243138005 0.0024772174699799845 0.0023786792654153892 0.0020316457847079574 0.0014650458441179052 0.00073198021892930624 -9.5165616451746313e-05 -0.00093179550640667356 -0.0016896353737900064 -0.002286029399938193 -0.0026528026156592069 -0.0027439824010879752 -0.0025413474050266682 -0.0020572239101028095 -0.0013341713539966283 -0.00044143094406244902 0.00053155699309554165 0.0014839255272411029 0.0023137406585026126 0.0029286981481292974 0.0032562467484617786 0.003251908926443922 0.0029049085085457831 0.0022404564981489922 0.0013182816267311918 0.00022746308219447748 -0.00092196135663783645 -0.0020099732300794516 -0.0029188826132397309 -0.0035458920722500759 -0.0038144882122502053 -0.0036834454103191363 -0.0031524540265802821 -0.0022636032725808913 -0.001098441233437557 0.00022918138522259228 0.0015840095633793522 0.0028228488017388279 0.0038094256961896428 0.0044290486254589569 0.0046015294833341713 0.0042909951378952392 0.0035113829579288443 0.002326900465678434 0.00084726356737852785 -0.00078210688654584614 -0.0023939506744333323 -0.0038159332671489276 -0.0048886091342003283 -0.0054827496552296451 -0.0055142584805278339 -0.0049549620495624256 -0.0038379957384760514 -0.0022570524748253273 -0.00035920054838253909 0.0016681240381698865 0.0036149620582436124 0.0052698289441135563 0.0064418143583644455 0.0069816111699239911 0.0067991979917402107 0.0058762117387505652 0.0042715432406493607 0.0021191551611802598 -0.00038190594776891601 -0.0029847547360424441 -0.0054177398262781288 -0.0074112614644437011 -0.0087258737465600832 -0.0091788423919074678 -0.0086664128929747897 -0.0071793804592940056 -0.004809945117289164 -0.0017488049914463934 0.0017278402015994767 0.0052806440695748677 0.0085371287675241395 ...(+5120 chars)]  InputProcessing=Columns as channels (frame based)
  Out : Outport
  wires:
  In/1 -> Generated Filter Block/1
  Generated Filter Block/1 -> Out/1
